simulink model "InnerTransition1_2018a"  (R2018a)
settings: Solver=VariableStepAuto  StartTime=0.0  StopTime=10.0  RelTol=1e-3
settings Model: Creator=apple  LastModifiedBy=apple
settings DataIOCC: ReturnWorkspaceOutputs=on
settings SFSimCC: SimUseLocalCustomCode=on
settings RTWCC: RTWUseLocalCustomCode=on

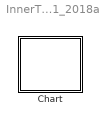
== system InnerTransition1_2018a ==
  Chart : Stateflow chart  TreatAsAtomicUnit=on

== stateflow chart InnerTransition1_2018a/Chart ==
  state A
    en:fprintf("Entry A");
    du:fprintf("During A");
    ex:fprintf("Exit A");
    A -> A [order 1] : /{fprintf("Transition Action2");}
  state B
    en:fprintf("Entry B");
    du:fprintf("During B");
    ex:fprintf("Exit B");
  (default) -> A : {x= 0;}
  A -> B [order 1] : E_one[x>0]/{fprintf("Transition Action1");}
  B -> A [order 1] : E_two[x>0]/{fprintf("Transition Action3");}
  B -> B [order 2] : /{fprintf("Transition Action4");}
  data: x local
  events: E_two local FUNCTION_CALL_EVENT; E_one local FUNCTION_CALL_EVENT
